simulink model "MFTiresLongitudinalFront"  (R2026b)
settings: Solver=VariableStepAuto
undefined symbols (not defined in the file): EnvGrvty, PlntVehDstCGFrntAxl, PlntVehDstCGRearAxl, PlntVehFzFlt, PlntVehMass, PlntWhlNumFrnt
libraries: autolibshared x2, simulink_extras x2
(part 2 of 2)

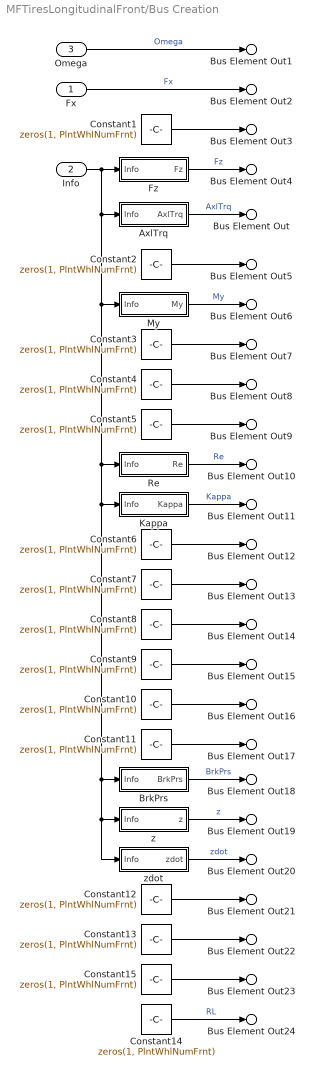
== system MFTiresLongitudinalFront/Bus Creation ==
  Fx : Inport
  Info : Inport  Port=2
  Omega : Inport  Port=3
  AxlTrq : Subsystem
  BrkPrs : Subsystem
  Constant{1..15} (15 alike) : Constant  Value=zeros(1, PlntWhlNumFrnt)  SampleTime=Inf
  Fz : Subsystem
  Kappa : Subsystem
  My : Subsystem
  Re : Subsystem
  z : Subsystem
  zdot : Subsystem
  Bus Element Out : Outport  PortName=Wheels  Element=AxlTrq
  Bus Element Out1 : Outport  PortName=Wheels  Element=Omega
  Bus Element Out2 : Outport  PortName=Wheels  Element=Fx
  Bus Element Out3 : Outport  PortName=Wheels  Element=Fy
  Bus Element Out4 : Outport  PortName=Wheels  Element=Fz
  Bus Element Out5 : Outport  PortName=Wheels  Element=Mx
  Bus Element Out6 : Outport  PortName=Wheels  Element=My
  Bus Element Out7 : Outport  PortName=Wheels  Element=Mz
  Bus Element Out8 : Outport  PortName=Wheels  Element=Vx
  Bus Element Out9 : Outport  PortName=Wheels  Element=Vy
  Bus Element Out10 : Outport  PortName=Wheels  Element=Re
  Bus Element Out24 : Outport  PortName=Wheels  Element=RL
  Bus Element Out11 : Outport  PortName=Wheels  Element=Kappa
  Bus Element Out12 : Outport  PortName=Wheels  Element=Alpha
  Bus Element Out13 : Outport  PortName=Wheels  Element=a
  Bus Element Out14 : Outport  PortName=Wheels  Element=b
  Bus Element Out15 : Outport  PortName=Wheels  Element=Gamma
  Bus Element Out16 : Outport  PortName=Wheels  Element=psidot
  Bus Element Out17 : Outport  PortName=Wheels  Element=BrkTrq
  Bus Element Out18 : Outport  PortName=Wheels  Element=BrkPrs
  Bus Element Out19 : Outport  PortName=Wheels  Element=z
  Bus Element Out20 : Outport  PortName=Wheels  Element=zdot
  Bus Element Out21 : Outport  PortName=Wheels  Element=Gnd
  Bus Element Out22 : Outport  PortName=Wheels  Element=GndFz
  Bus Element Out23 : Outport  PortName=Wheels  Element=Prs
  wires:
  AxlTrq/1(AxlTrq) -> Bus Element Out/1  "AxlTrq"
  Constant15/1 -> Bus Element Out23/1
  Constant13/1 -> Bus Element Out22/1
  Constant12/1 -> Bus Element Out21/1
  Constant11/1 -> Bus Element Out17/1
  Constant10/1 -> Bus Element Out16/1
  Constant9/1 -> Bus Element Out15/1
  Constant8/1 -> Bus Element Out14/1
  Constant7/1 -> Bus Element Out13/1
  Constant6/1 -> Bus Element Out12/1
  Constant5/1 -> Bus Element Out9/1
  Constant4/1 -> Bus Element Out8/1
  Constant3/1 -> Bus Element Out7/1
  Constant1/1 -> Bus Element Out3/1
  Constant2/1 -> Bus Element Out5/1
  Fx/1 -> Bus Element Out2/1  "Fx"
  Omega/1 -> Bus Element Out1/1  "Omega"
  Fz/1(Fz) -> Bus Element Out4/1  "Fz"
  Info/1 -> zdot/1(Info), z/1(Info), BrkPrs/1(Info), Kappa/1(Info), Re/1(Info), My/1(Info), AxlTrq/1(Info), Fz/1(Info)
  My/1(My) -> Bus Element Out6/1  "My"
  Re/1(Re) -> Bus Element Out10/1  "Re"
  Kappa/1(Kappa) -> Bus Element Out11/1  "Kappa"
  BrkPrs/1(BrkPrs) -> Bus Element Out18/1  "BrkPrs"
  z/1(z) -> Bus Element Out19/1  "z"
  zdot/1(zdot) -> Bus Element Out20/1  "zdot"
  Constant14/1 -> Bus Element Out24/1  "RL"

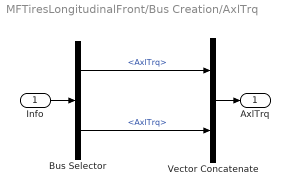
== system MFTiresLongitudinalFront/Bus Creation/AxlTrq ==
  Info : Inport
  Bus Selector : BusSelector  OutputSignals=L.AxlTrq,R.AxlTrq
  Vector Concatenate : Concatenate
  AxlTrq : Outport  VectorParamsAs1DForOutWhenUnconnected=off
  wires:
  Bus Selector/2 -> Vector Concatenate/2  "<AxlTrq>"
  Bus Selector/1 -> Vector Concatenate/1  "<AxlTrq>"
  Vector Concatenate/1 -> AxlTrq/1
  Info/1 -> Bus Selector/1

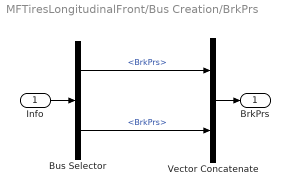
== system MFTiresLongitudinalFront/Bus Creation/BrkPrs ==
  Info : Inport
  Bus Selector : BusSelector  OutputSignals=L.BrkPrs,R.BrkPrs
  Vector Concatenate : Concatenate
  BrkPrs : Outport  VectorParamsAs1DForOutWhenUnconnected=off
  wires:
  Vector Concatenate/1 -> BrkPrs/1
  Info/1 -> Bus Selector/1
  Bus Selector/2 -> Vector Concatenate/2  "<BrkPrs>"
  Bus Selector/1 -> Vector Concatenate/1  "<BrkPrs>"

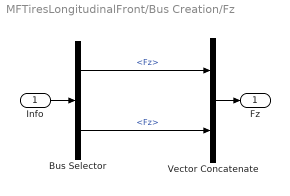
== system MFTiresLongitudinalFront/Bus Creation/Fz ==
  Info : Inport
  Bus Selector : BusSelector  OutputSignals=L.Fz,R.Fz
  Vector Concatenate : Concatenate
  Fz : Outport  VectorParamsAs1DForOutWhenUnconnected=off
  wires:
  Info/1 -> Bus Selector/1
  Vector Concatenate/1 -> Fz/1
  Bus Selector/1 -> Vector Concatenate/1  "<Fz>"
  Bus Selector/2 -> Vector Concatenate/2  "<Fz>"

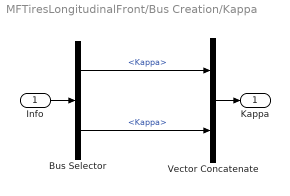
== system MFTiresLongitudinalFront/Bus Creation/Kappa ==
  Info : Inport
  Bus Selector : BusSelector  OutputSignals=L.Kappa,R.Kappa
  Vector Concatenate : Concatenate
  Kappa : Outport  VectorParamsAs1DForOutWhenUnconnected=off
  wires:
  Bus Selector/1 -> Vector Concatenate/1  "<Kappa>"
  Bus Selector/2 -> Vector Concatenate/2  "<Kappa>"
  Info/1 -> Bus Selector/1
  Vector Concatenate/1 -> Kappa/1

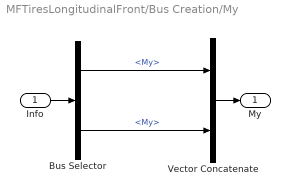
== system MFTiresLongitudinalFront/Bus Creation/My ==
  Info : Inport
  Bus Selector : BusSelector  OutputSignals=L.My,R.My
  Vector Concatenate : Concatenate
  My : Outport  VectorParamsAs1DForOutWhenUnconnected=off
  wires:
  Info/1 -> Bus Selector/1
  Vector Concatenate/1 -> My/1
  Bus Selector/1 -> Vector Concatenate/1  "<My>"
  Bus Selector/2 -> Vector Concatenate/2  "<My>"

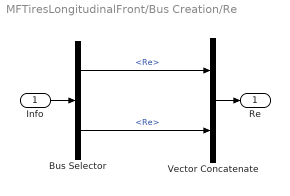
== system MFTiresLongitudinalFront/Bus Creation/Re ==
  Info : Inport
  Bus Selector : BusSelector  OutputSignals=L.Re,R.Re
  Vector Concatenate : Concatenate
  Re : Outport  VectorParamsAs1DForOutWhenUnconnected=off
  wires:
  Bus Selector/1 -> Vector Concatenate/1  "<Re>"
  Bus Selector/2 -> Vector Concatenate/2  "<Re>"
  Info/1 -> Bus Selector/1
  Vector Concatenate/1 -> Re/1

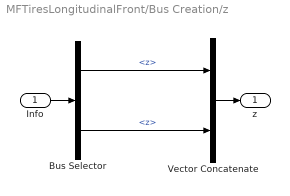
== system MFTiresLongitudinalFront/Bus Creation/z ==
  Info : Inport
  Bus Selector : BusSelector  OutputSignals=L.z,R.z
  Vector Concatenate : Concatenate
  z : Outport  VectorParamsAs1DForOutWhenUnconnected=off
  wires:
  Bus Selector/1 -> Vector Concatenate/1  "<z>"
  Bus Selector/2 -> Vector Concatenate/2  "<z>"
  Info/1 -> Bus Selector/1
  Vector Concatenate/1 -> z/1

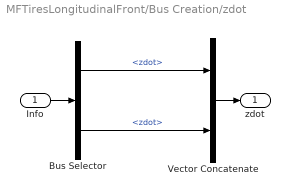
== system MFTiresLongitudinalFront/Bus Creation/zdot ==
  Info : Inport
  Bus Selector : BusSelector  OutputSignals=L.zdot,R.zdot
  Vector Concatenate : Concatenate
  zdot : Outport  VectorParamsAs1DForOutWhenUnconnected=off
  wires:
  Vector Concatenate/1 -> zdot/1
  Info/1 -> Bus Selector/1
  Bus Selector/2 -> Vector Concatenate/2  "<zdot>"
  Bus Selector/1 -> Vector Concatenate/1  "<zdot>"
